simulink model "task2_pos"  (R2024b)
settings: Solver=VariableStepAuto  StartTime=0.0  StopTime=stop_time  RelTol=1e-3
values from neighbouring files (symbols this model uses):
  p_0 = [17, 22.5, 0]'    [MAIN.m]    (also in MAIN_exam_2025.m = [0 0 0]')
  UAV = include_pack(UAV,pack,1)    [MAIN.m]
  vb_0 = zeros(3,1)    [MAIN.m]    (also in MAIN_exam_2025.m = [0 0 0]')
undefined symbols (not defined in the file or in its folder): ctrl, par
settings Model: Creator=invernizzi  LastModifiedBy=ggera

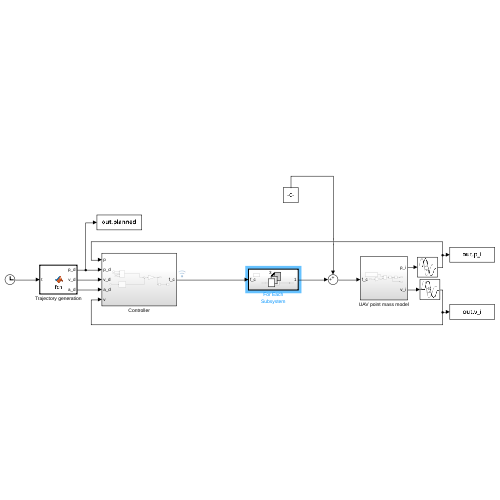
[thumbnail: Simulink's stored preview of the top-level diagram]
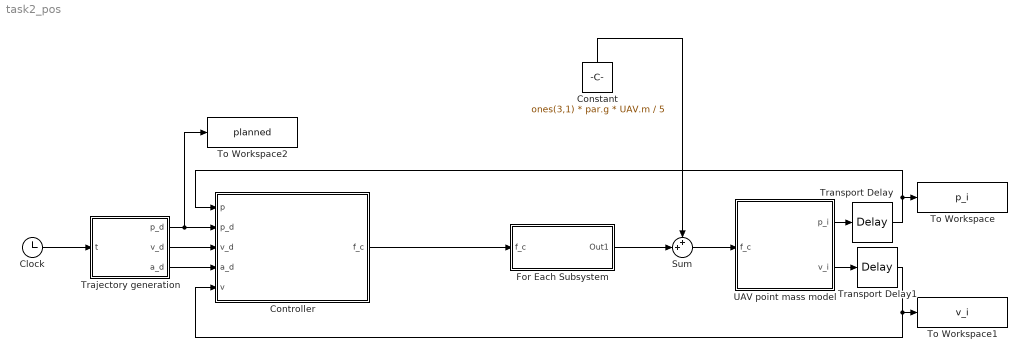
== system task2_pos ==
  Clock : Clock
  Constant : Constant  Value=ones(3,1) * par.g * UAV.m / 5
  Controller : Subsystem
  For Each Subsystem : Subsystem  TreatAsAtomicUnit=on
  Sum : Sum  Inputs=++|
  To Workspace : ToWorkspace  VariableName=p_i  SaveFormat=Timeseries  SampleTime=-1
  To Workspace1 : ToWorkspace  VariableName=v_i  SaveFormat=Timeseries  SampleTime=-1
  To Workspace2 : ToWorkspace  VariableName=planned  SaveFormat=Timeseries  SampleTime=-1
  Trajectory generation : MATLAB Function  TreatAsAtomicUnit=on
  Transport Delay : TransportDelay  DelayTime=0.03
  Transport Delay1 : TransportDelay  DelayTime=0.03
  UAV point mass model : Subsystem
  wires:
  UAV point mass model/2(v_i) -> Transport Delay1/1
  Clock/1 -> Trajectory generation/1(t)
  UAV point mass model/1(p_i) -> Transport Delay/1
  Trajectory generation/1(p_d) -> Controller/2(p_d), To Workspace2/1
  Trajectory generation/2(v_d) -> Controller/3(v_d)
  Trajectory generation/3(a_d) -> Controller/4(a_d)
  Sum/1 -> UAV point mass model/1(f_c)
  Constant/1 -> Sum/1
  For Each Subsystem/1(Out1) -> Sum/2
  Controller/1(f_c) -> For Each Subsystem/1(f_c)
  Transport Delay/1 -> Controller/1(p), To Workspace/1
  Transport Delay1/1 -> Controller/5(v), To Workspace1/1

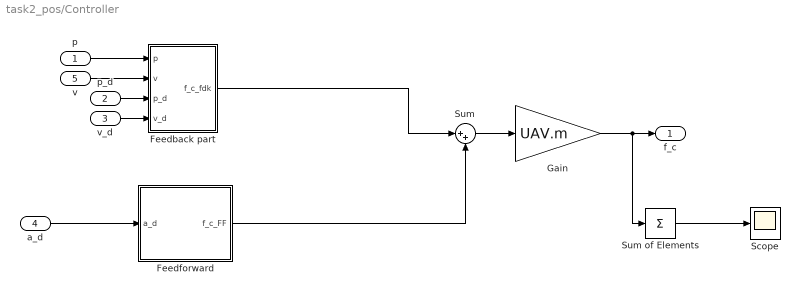
== system task2_pos/Controller ==
  p : Inport
  p_d : Inport  Port=2
  v_d : Inport  Port=3
  a_d : Inport  Port=4
  v : Inport  Port=5
  Feedback part : Subsystem
  Feedforward : Subsystem
  Gain : Gain  Gain=UAV.m
  Scope : Scope
  Sum : Sum  Inputs=|++
  Sum of Elements : Sum  Inputs=+
  f_c : Outport
  wires:
  Feedback part/1(f_c_fdk) -> Sum/1
  v_d/1 -> Feedback part/4(v_d)
  Feedforward/1(f_c_FF) -> Sum/2
  a_d/1 -> Feedforward/1(a_d)
  v/1 -> Feedback part/2(v)
  p_d/1 -> Feedback part/3(p_d)
  Sum/1 -> Gain/1
  p/1 -> Feedback part/1(p)
  Gain/1 -> Sum of Elements/1, f_c/1
  Sum of Elements/1 -> Scope/1

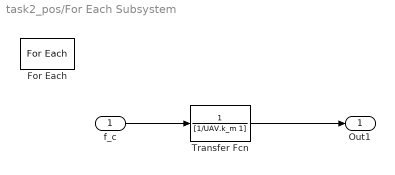
== system task2_pos/For Each Subsystem ==
  f_c : Inport  Partition=on  PartitionDimension=1  PartitionWidth=1  PartitionOffset=0
  For Each : ForEach  DisableCoverage=on
  Transfer Fcn : TransferFcn  Denominator=[1/UAV.k_m 1]
  Out1 : Outport  ConcatenationDimension=1
  wires:
  f_c/1 -> Transfer Fcn/1
  Transfer Fcn/1 -> Out1/1

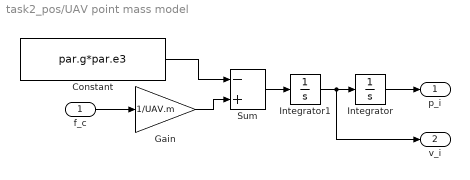
== system task2_pos/UAV point mass model ==
  f_c : Inport
  Constant : Constant  Value=par.g*par.e3
  Gain : Gain  Gain=1/UAV.m
  Integrator : Integrator  InitialCondition=p_0
  Integrator1 : Integrator  InitialCondition=vb_0
  Sum : Sum  Inputs=-+
  p_i : Outport
  v_i : Outport  Port=2
  wires:
  f_c/1 -> Gain/1
  Gain/1 -> Sum/2
  Constant/1 -> Sum/1
  Integrator/1 -> p_i/1
  Integrator1/1 -> v_i/1, Integrator/1
  Sum/1 -> Integrator1/1

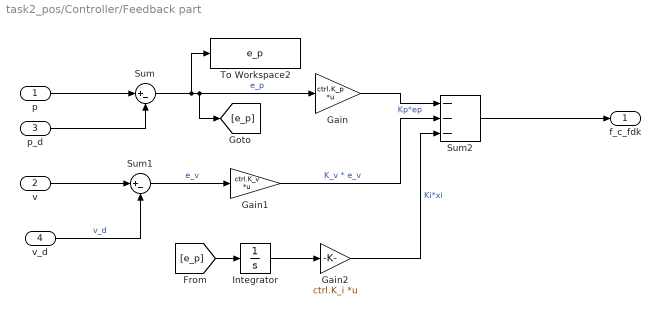
== system task2_pos/Controller/Feedback part ==
  p : Inport
  v : Inport  Port=2
  p_d : Inport  Port=3
  v_d : Inport  Port=4
  Gain : Gain  Gain=ctrl.K_p  Multiplication=Matrix(K*u)
  Gain1 : Gain  Gain=ctrl.K_v  Multiplication=Matrix(K*u)
  Gain2 : Gain  Gain=ctrl.K_i  Multiplication=Matrix(K*u)
  Integrator : Integrator
  Sum : Sum  Inputs=|+-
  Sum1 : Sum  Inputs=|+-
  Sum2 : Sum  Inputs=---
  To Workspace2 : ToWorkspace  VariableName=e_p  SaveFormat=Timeseries  SampleTime=-1
  f_c_fdk : Outport
  wires:
  p_d/1 -> Sum/2
  v/1 -> Sum1/1
  Gain1/1 -> Sum2/2  "K_v * e_v"
  Sum1/1 -> Gain1/1  "e_v"
  v_d/1 -> Sum1/2  "v_d"
  Sum2/1 -> f_c_fdk/1
  p/1 -> Sum/1
  Gain/1 -> Sum2/1  "Kp*ep"
  Sum/1 -> To Workspace2/1, [e_p], Gain/1  "e_p"
  Integrator/1 -> Gain2/1
  Gain2/1 -> Sum2/3  "Ki*xi"
  [e_p] -> Integrator/1

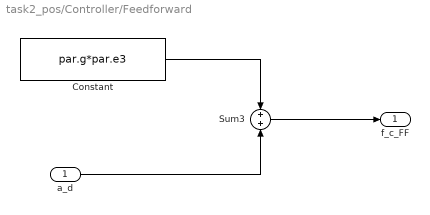
== system task2_pos/Controller/Feedforward ==
  a_d : Inport
  Constant : Constant  Value=par.g*par.e3
  Sum3 : Sum
  f_c_FF : Outport
  wires:
  Constant/1 -> Sum3/1
  a_d/1 -> Sum3/2
  Sum3/1 -> f_c_FF/1

== matlab function task2_pos/Trajectory generation ==
  data: t input; p_d output; v_d output; a_d output
function [p_d,v_d,a_d] = fcn(t)

%setpoint tracking
Omega_d=1; % rad/s
R_d=1; % m

p_d = R_d*[cos(Omega_d*t) sin(Omega_d*t) 1]';
v_d = R_d*Omega_d*[-sin(Omega_d*t) cos(Omega_d*t) 0]';
a_d = -R_d*Omega_d^2*[cos(Omega_d*t) sin(Omega_d*t) 0]';

% p_d = [1 1 1]';
% v_d = zeros(3,1);
% a_d = v_d;
